simulink model "quadrotorsmodel1"  (R2025b)
settings: Solver=FixedStepAuto  StartTime=0.0  StopTime=SimulationTime  FixedStep=timestep  RelTol=1e-3
values from neighbouring files (symbols this model uses):
  g = 9.81    [fak.m]
  I = eye(3,3)    [fak.m]
  K = [1 1 1 1 ... (first row only)    [fak.m]
  m = 4.34    [fak.m]    (also in min_snap_Coef.m = length(timepoints) - 1)
settings Model: Creator=worap  LastModifiedBy=IXVIA
settings DataIOCC: ExternalInput=inputStructure  LoadExternalInput=on

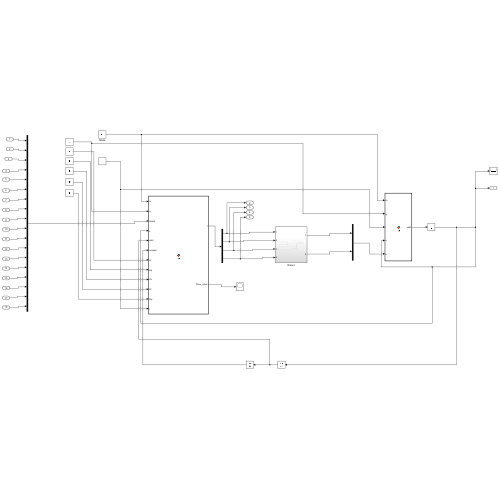
[thumbnail: Simulink's stored preview of the top-level diagram]
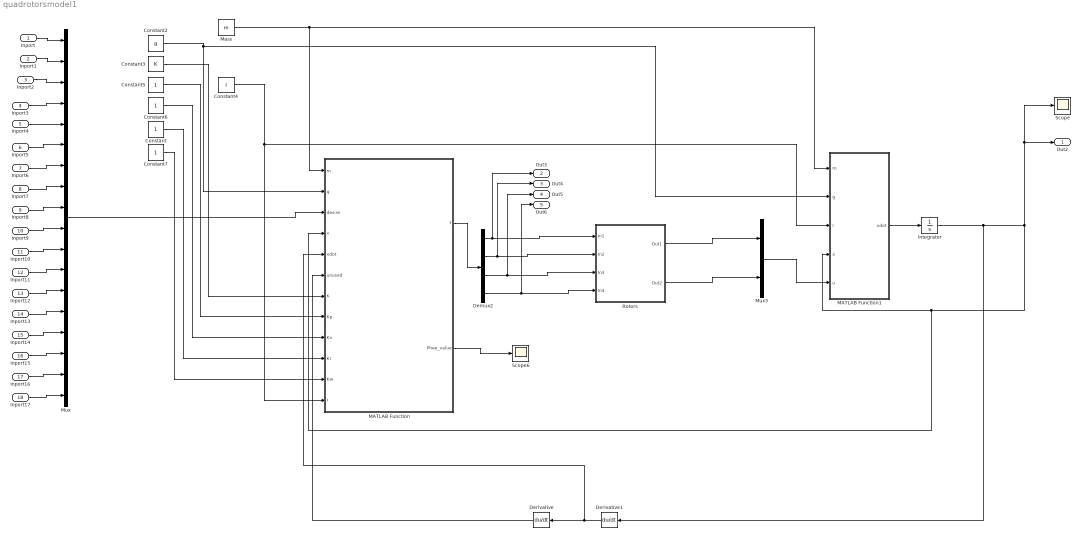
== system quadrotorsmodel1 ==
  Inport : Inport
  Inport1 : Inport  Port=2
  Inport2 : Inport  Port=3
  Inport3 : Inport  Port=4
  Inport4 : Inport  Port=5
  Inport5 : Inport  Port=6
  Inport6 : Inport  Port=7
  Inport7 : Inport  Port=8
  Inport8 : Inport  Port=9
  Inport9 : Inport  Port=10
  Inport10 : Inport  Port=11
  Inport11 : Inport  Port=12
  Inport12 : Inport  Port=13
  Inport13 : Inport  Port=14
  Inport14 : Inport  Port=15
  Inport15 : Inport  Port=16
  Inport16 : Inport  Port=17
  Inport17 : Inport  Port=18
  Constant{,5..7} (4 alike) : Constant
  Constant2 : Constant  Value=g
  Constant3 : Constant  Value=K
  Constant4 : Constant  Value=I
  Demux2 : Demux
  Derivative : Derivative
  Derivative1 : Derivative
  Integrator : Integrator  InitialCondition=[0;0;0;0;0;0;1;0;0;0;1;0;0;0;1;0;0;0]
  MATLAB Function : MATLAB Function  TreatAsAtomicUnit=on
  MATLAB Function1 : MATLAB Function  TreatAsAtomicUnit=on
  Mass : Constant  Value=m
  Mux : Mux  Inputs=18
  Mux3 : Mux  Inputs=2
  Rotors : Subsystem
  Scope : Scope
      settings: ActiveDisplayYMinimum=-1478.5838254344892  ActiveDisplayYMaximum=2676.5749852449244
  Scope6 : Scope
      settings: ActiveDisplayYMinimum=-0.10349  ActiveDisplayYMaximum=2.21622
  Out2 : Outport
  Out3 : Outport  Port=2
  Out4 : Outport  Port=3
  Out5 : Outport  Port=4
  Out6 : Outport  Port=5
  wires:
  Mass/1 -> MATLAB Function1/1(m), MATLAB Function/1(m)
  Demux2/2 -> Out4/1, Rotors/2(In2)
  Rotors/1(Out1) -> Mux3/1
  Rotors/2(Out2) -> Mux3/2
  Demux2/3 -> Out5/1, Rotors/3(In3)
  Demux2/4 -> Out6/1, Rotors/4(In4)
  Constant4/1 -> MATLAB Function1/3(I), MATLAB Function/12(I)
  MATLAB Function/1(f) -> Demux2/1
  Demux2/1 -> Out3/1, Rotors/1(In1)
  Constant2/1 -> MATLAB Function1/2(g), MATLAB Function/2(g)
  Constant3/1 -> MATLAB Function/7(K)
  Constant5/1 -> MATLAB Function/8(Kp)
  Constant6/1 -> MATLAB Function/9(Kv)
  Constant7/1 -> MATLAB Function/11(Kw)
  Constant/1 -> MATLAB Function/10(Kr)
  MATLAB Function/2(Phee_value) -> Scope6/1
  Mux3/1 -> MATLAB Function1/5(u)
  MATLAB Function1/1(xdot) -> Integrator/1
  Integrator/1 -> Derivative1/1, MATLAB Function/4(x), MATLAB Function1/4(x), Scope/1, Out2/1
  Mux/1 -> MATLAB Function/3(desire)
  Inport17/1 -> Mux/18
  Inport16/1 -> Mux/17
  Inport15/1 -> Mux/16
  Inport14/1 -> Mux/15
  Inport13/1 -> Mux/14
  Inport12/1 -> Mux/13
  Inport11/1 -> Mux/12
  Inport10/1 -> Mux/11
  Inport9/1 -> Mux/10
  Inport8/1 -> Mux/9
  Inport7/1 -> Mux/8
  Inport6/1 -> Mux/7
  Inport5/1 -> Mux/6
  Inport4/1 -> Mux/5
  Inport3/1 -> Mux/4
  Inport2/1 -> Mux/3
  Inport1/1 -> Mux/2
  Inport/1 -> Mux/1
  Derivative/1 -> MATLAB Function/6(unused)
  Derivative1/1 -> MATLAB Function/5(xdot), Derivative/1

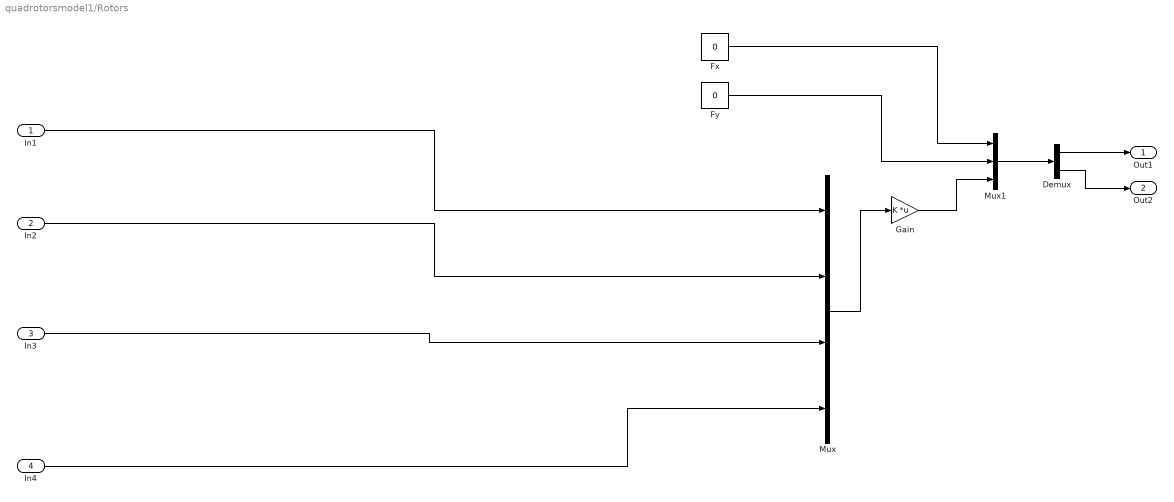
== system quadrotorsmodel1/Rotors ==
  In1 : Inport
  In2 : Inport  Port=2
  In3 : Inport  Port=3
  In4 : Inport  Port=4
  Demux : Demux  Outputs=2
  Fx : Constant  Value=0
  Fy : Constant  Value=0
  Gain : Gain  Gain=K  Multiplication=Matrix(K*u) (u vector)
  Mux : Mux
  Mux1 : Mux  Inputs=3
  Out1 : Outport
  Out2 : Outport  Port=2
  wires:
  Fx/1 -> Mux1/1
  Mux1/1 -> Demux/1
  Fy/1 -> Mux1/2
  Mux/1 -> Gain/1
  Gain/1 -> Mux1/3
  Demux/2 -> Out2/1
  Demux/1 -> Out1/1
  In1/1 -> Mux/1
  In2/1 -> Mux/2
  In3/1 -> Mux/3
  In4/1 -> Mux/4

== matlab function quadrotorsmodel1/MATLAB Function1 ==
  data: m input; g input; I input; x input; u input; xdot output
function xdot = fcn(m,g,I,x,u)

% extract the x-vextor
p = x(1:3,1);
v = x(4:6,1);
R = reshape(x(7:15,1),3,3);
omega = x(16:18,1);

%control signal
f = u(3,1);
M = u(4:6,1);

e3 = [0;0;1];


xdot = zeros(size(x));

xdot(1:3,1) = v;
xdot(4:6,1) = g*e3 - 1/m*f*R*e3;

Rdot = R*hatmap(omega);
xdot(7:15,1) = Rdot(:);

xdot(16:18,1) = I\(M - cross(omega,I*omega));




end

== matlab function quadrotorsmodel1/MATLAB Function ==
  data: m input; g input; f output; Phee_value output; desire input; x input; xdot input; unused input; K input; Kp input; Kv input; Kr input; Kw input; I input
function [f, Phee_value] = fcn(m, g, desire, x, xdot, ~, K, Kp, Kv, Kr, Kw, I)
%#codegen

% ---- preallocate outputs (fix dims) ----
f = zeros(4,1);
Phee_value = 0;

e3 = [0;0;1];


% -------- desired --------
rd    = desire(1:3);
vd    = desire(4:6);
ad    = desire(7:9);
jd    = desire(10:12);    
psid  = desire(16);
dpsid = desire(17);

% -------- actual --------
p     = x(1:3);
v     = xdot(1:3);
R     = reshape(x(7:15),3,3);
omega = x(16:18);

phi = atan2(R(3,2), R(3,3));
Phee_value = phi;

% -------- gains --------
if isempty(I), I = eye(3); end
Ix = I(1,1); Iy = I(2,2); Iz = I(3,3);

Kp = diag([4.0*m, 4.0*m, 12.0*m]);
Kv = diag([8.0*m, 8.0*m, 10.0*m]);
Kr = diag([(8.0^2)*Ix, (8.0^2)*Iy, (5.5^2)*Iz]);
Kw = diag([2*8.0*Ix,   2*8.0*Iy,   2*5.5*Iz]);

% -------- force with feedforward --------
dt = 0.01;                       % ให้ตรงกับ sample time ของบล็อก
jerk_ff = 0;

vel_error_magnitude = norm(v - vd);
vel_ff_gain = min(0.25, norm(v - vd) / 4.0);
vel_ff = vel_ff_gain * m * (ad - [0;0;g]);

A = -Kp*(p-rd) - Kv*(v-vd) - m*g*e3 + m*ad + jerk_ff + vel_ff;

A_norm = norm(A);
if A_norm < 1e-9
    A = -m*g*e3; A_norm = m*g;
end

% -------- desired attitude --------
b3c = -A / A_norm;
cpsi = cos(psid); spsi = sin(psid);
b1d  = [cpsi; spsi; 0];
b2c  = cross(b3c,b1d); nb2 = norm(b2c);
if nb2 < 1e-9
    b1d=[cpsi;spsi;1e-3]; b2c=cross(b3c,b1d); nb2=norm(b2c);
    if nb2 < 1e-12, nb2 = 1e-12; end
end
b2c = b2c/nb2;  b1c = cross(b2c,b3c);
Rc  = [b1c,b2c,b3c];

% -------- attitude errors --------
eR_mat = 0.5*(Rc.'*R - R.'*Rc);
eR = [eR_mat(3,2); eR_mat(1,3); eR_mat(2,1)];
eOmega = omega - (R.'*Rc)*[0;0;dpsid];

% -------- thrust & moments --------
Re3 = R*e3;
T = -A.'*Re3;
M = -Kr*eR - Kw*eOmega;

% thrust & moment limits
if ~isfinite(T), T = m*g; end
T = max(0.05*m*g, min(T, 3.5*m*g));

M_max = [1.0; 1.0; 0.4];
for i=1:3
    if ~isfinite(M(i)), M(i)=0; end
    M(i) = max(-M_max(i), min(M(i), M_max(i)));
end

% -------- allocation --------
U = [T; M];
omega2 = K \ U;
f = omega2;

end
